simulink model "L1_3"  (Simulink 7.9)
settings: Solver=ode45  StartTime=0.0  StopTime=1.5  RelTol=1e-3
libraries: simulink x1
settings Model: Creator=Павло  LastModifiedBy=Павло

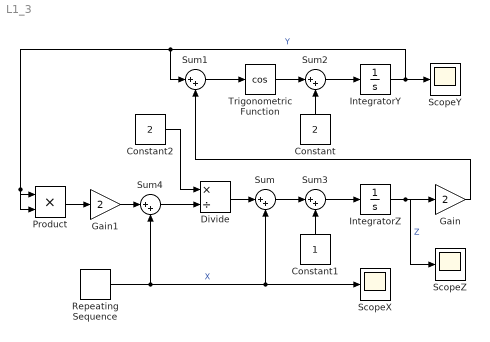
== system L1_3 ==
  Constant : Constant  Value=2
  Constant1 : Constant
  Constant2 : Constant  Value=2
  Divide : Product  Inputs=*/
  Gain : Gain  Gain=2
  Gain1 : Gain  Gain=2
  IntegratorY : Integrator  InitialCondition=1
  IntegratorZ : Integrator  InitialCondition=0.05
  Product : Product  RndMeth=Zero
  Repeating Sequence : simulink/Sources/Repeating Sequence  rep_seq_t=[0 4]  rep_seq_y=[0 4]
  ScopeX : Scope
      settings: TickLabels=on  TimeRange=0.9379378758757522  YMin=0.2922020202020199  YMax=0.54820202020202  SaveName=ScopeData2
  ScopeY : Scope
  ScopeZ : Scope
      settings: TickLabels=on  TimeRange=0.9379378758757522  YMin=0.2922020202020199  YMax=0.54820202020202
  Sum{,1..4} (5 alike) : Sum  Inputs=|++
  Trigonometric Function : Trigonometry  Operator=cos
  wires:
  IntegratorZ/1 -> ScopeZ/1, Gain/1  "Z"
  IntegratorY/1 -> ScopeY/1, Sum1/1, Product/2, Product/1  "Y"
  Sum2/1 -> IntegratorY/1
  Sum3/1 -> IntegratorZ/1
  Repeating Sequence/1 -> Sum4/2, ScopeX/1, Sum/2  "X"
  Constant/1 -> Sum2/2
  Constant1/1 -> Sum3/2
  Sum/1 -> Sum3/1
  Trigonometric Function/1 -> Sum2/1
  Sum1/1 -> Trigonometric Function/1
  Gain/1 -> Sum1/2
  Divide/1 -> Sum/1
  Constant2/1 -> Divide/1
  Sum4/1 -> Divide/2
  Gain1/1 -> Sum4/1
  Product/1 -> Gain1/1
